simulink model "obliczeniaOffline (1)"  (R2013a)
settings: Solver=FixedStepDiscrete  StartTime=0  StopTime=15  FixedStep=0.0025  RelTol=1e-3
InitFcn:
  | InitFcn
values from neighbouring files (symbols this model uses):
  accBias = zeros(3,1)    [InitFcn.m]
  accGain = accGain.*(9.81/9.761)    [InitFcn.m]
  gyroBias = zeros(3,1)    [InitFcn.m]
  gyroGain = ones(3,1)    [InitFcn.m]
  index = 1    [InitFcn.m]
  magBias = [(743-502);(743-507);(579-516)]/2    [InitFcn.m]
  magGainM = W_inverted    [InitFcn.m]
  usrednien = 5    [InitFcn.m]
undefined symbols (not defined in the file or in its folder): dfilt, DiscIntNeverNeededParam, eul_0, fdesignblkfcn, gcbh
libraries: dspstat3 x12, aerolibconvert2 x9, aerolibobsolete x7, aerolibtransform2 x4, dsparch4 x3, dspmtrx3 x3, aerolibutil x3, dspsigops x1, dspsrcs4 x1
(part 2 of 2)

== system obliczeniaOffline (1)/Euler z żyrskopu - całkowanie/Calculate Euler ==
  p q r : Inport
  reset : Inport  Port=2
  initialAngles : Inport  Port=3
  Discrete-Time Integrator1 : DiscreteIntegrator  ExternalReset=either  InitialConditionSource=external  InitialCondition=eul_0  SampleTime=-1  ICPrevOutput=DiscIntNeverNeededParam  ICPrevScaledInput=DiscIntNeverNeededParam
  phidot thetadot psidot : Subsystem
  Euler : Outport
  wires:
  p q r/1 -> phidot thetadot psidot/1(p q r)
  phidot thetadot psidot/1(phidot thetadot psi) -> Discrete-Time Integrator1/1
  Discrete-Time Integrator1/1 -> phidot thetadot psidot/2(phi theta psi), Euler/1
  reset/1 -> Discrete-Time Integrator1/2
  initialAngles/1 -> Discrete-Time Integrator1/3

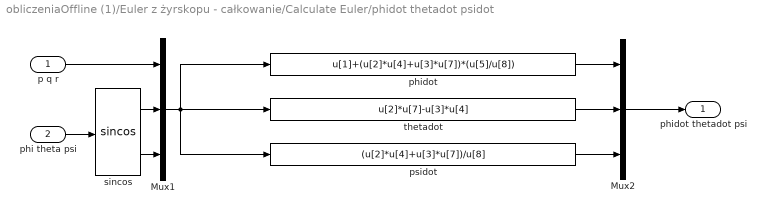
== system obliczeniaOffline (1)/Euler z żyrskopu - całkowanie/Calculate Euler/phidot thetadot psidot ==
  p q r : Inport
  phi theta psi : Inport  Port=2
  Mux1 : Mux  Inputs=[3 3 3]
  Mux2 : Mux  Inputs=3
  phidot : Fcn  Expr=u[1]+(u[2]*u[4]+u[3]*u[7])*(u[5]/u[8])
  psidot : Fcn  Expr=(u[2]*u[4]+u[3]*u[7])/u[8]
  sincos : Trigonometry  Operator=sincos
  thetadot : Fcn  Expr=u[2]*u[7]-u[3]*u[4]
  phidot thetadot psi : Outport  InitialOutput=0
  wires:
  phi theta psi/1 -> sincos/1
  psidot/1 -> Mux2/3
  thetadot/1 -> Mux2/2
  sincos/1 -> Mux1/2
  p q r/1 -> Mux1/1
  sincos/2 -> Mux1/3
  Mux2/1 -> phidot thetadot psi/1
  phidot/1 -> Mux2/1
  Mux1/1 -> phidot/1, psidot/1, thetadot/1
